simulink model "SMC_Boost4"  (R2016b)
settings: Solver=VariableStepAuto  StartTime=0.0  StopTime=0.1  RelTol=1e-3
libraries: powerlib x13
settings Model: Creator=mahdi  LastModifiedBy=mahdi

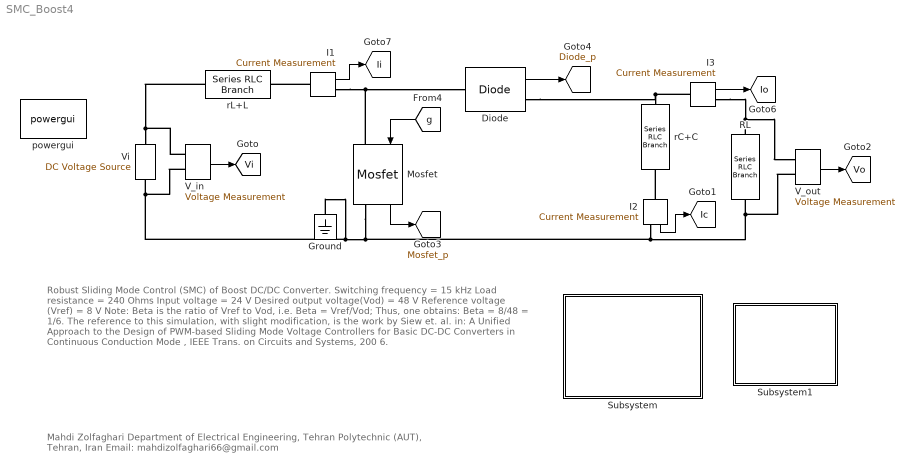
== system SMC_Boost4 ==
  note: Mahdi Zolfaghari
      | Department of Electrical Engineering, Tehran Polytechnic (AUT), Tehran, Iran
      | Email: mahdizolfaghari66@gmail.com
  note: Robust Sliding Mode Control (SMC) of Boost DC/DC Converter.
      | Switching frequency = 15 kHz
      | Load resistance = 240 Ohms
      | Input voltage = 24 V
      | Desired output voltage(Vod) = 48 V
      | Reference voltage (Vref) = 8 V
      | Note: Beta is the ratio of Vref to Vod, i.e. Beta = Vref/Vod; Thus, one obtains:
      | Beta = 8/48 = 1/6.
      | The reference to this simulation, with slight modification, is the work by Siew et. al. in:
      | A Unified Approach to the Design of PWM-based Sliding Mode Voltage Controllers
      | for Basic DC-DC Converters in Continuous Conduction Mode , IEEE Trans. on Circuits and Systems, 200 6.
  Diode : powerlib/Power Electronics/Diode  Ron=0.001  Lon=0  Vf=0.8  IC=0  UseSnubber=off  Rs=500  Cs=250e-9  Measurements=on
  Ground : powerlib/Elements/Ground  LConnTagsString=a
  I1 : powerlib/Measurements/Current Measurement  PhasorSimulation=off  OutputType=Complex  PSBequivalent=0
  I2 : powerlib/Measurements/Current Measurement  PhasorSimulation=off  OutputType=Complex  PSBequivalent=0
  I3 : powerlib/Measurements/Current Measurement  PhasorSimulation=off  OutputType=Complex  PSBequivalent=0
  Mosfet : powerlib/Power Electronics/Mosfet  Ron=0.1  Lon=0  Rd=0.01  Vfd=0  IC=0  Rs=1e5  Cs=inf  Measurements=on
  RL : powerlib/Elements/Series RLC Branch  LConnTagsString=__new0  RConnTagsString=__new0  BranchType=R  Resistance=240  Inductance=1e-3  SetiL0=off  InitialCurrent=0  Capacitance=0  Setx0=off  InitialVoltage=0  Measurements=None
  Subsystem : Subsystem
      mask Display: disp('Sliding Mode\nController')
  Subsystem1 : Subsystem
      mask Display: disp('Measurements')
  V_in : powerlib/Measurements/Voltage Measurement  PhasorSimulation=off  OutputType=Complex  PSBequivalent=0
  V_out : powerlib/Measurements/Voltage Measurement  PhasorSimulation=off  OutputType=Complex  PSBequivalent=0
  Vi : powerlib/Electrical Sources/DC Voltage Source  Amplitude=24  Measurements=None
  powergui : powerlib/powergui  Priority=1  SimulationMode=Discrete  SolverType=Tustin/Backward Euler (TBE)  SampleTime=50e-6  frequency=60  SPID=off  DisableSnubberDevices=off  DisableRonSwitches=off  DisableVfSwitches=off  SwTol=0  DisplayEquations=off  Interpol=off  ExternalGateDelay=off  methode=off  Ts=10  FunctionMessages=off  echomessages=off  HookPort=off  EnableUseOfTLC=off  x0status=blocks  frequencyindice=0  Pbase=100e6  ErrMax=1e-4  Iterations=50  UnitsV=kV  UnitsW=MW  buscounter=0  RestoreLinks=warning  ResistiveCurrentMeasurement=off  Frange=[0:2:500]  Ylog=off  Xlog=on  ShowGrid=off  save=off  variable=ZData  structure=0  ZoomFFT=off  StartTime=0.0  cycles=1  DisplayStyle=1  fundamental=60  FreqAxis=off  MaxFrequency=1000  frequencyindicesteady=1  RmsSteady=1  display=off
  rC+C : powerlib/Elements/Series RLC Branch  LConnTagsString=__new0  RConnTagsString=__new0  BranchType=RC  Resistance=69e-3  Inductance=1e-3  SetiL0=off  InitialCurrent=0  Capacitance=2300e-6  Setx0=off  InitialVoltage=0  Measurements=None
  rL+L : powerlib/Elements/Series RLC Branch  LConnTagsString=__new0  RConnTagsString=__new0  BranchType=RL  Resistance=0.14  Inductance=300e-6  SetiL0=off  InitialCurrent=0  Capacitance=0  Setx0=off  InitialVoltage=0  Measurements=None
  tag scope: Diode_p=global, Ic=global, Ii=global, Io=global, Mosfet_p=global, Vi=global, Vo=global
  wires:
  V_out/1 -> [Vo]
  I2/1 -> [Ic]
  V_in/1 -> [Vi]
  [g] -> Mosfet/1
  Mosfet/1 -> [Mosfet_p]
  Diode/1 -> [Diode_p]
  I3/1 -> [Io]
  I1/1 -> [Ii]
  connections:
  I2/LConn1 -- rC+C/RConn1
  RL/LConn1 -- I3/RConn1 -- V_out/LConn1
  rL+L/LConn1 -- V_in/LConn1 -- Vi/RConn1
  I2/RConn1 -- Ground/LConn1 -- V_in/LConn2 -- Vi/LConn1 -- Mosfet/RConn1 -- V_out/LConn2 -- RL/RConn1
  Diode/RConn1 -- rC+C/LConn1 -- I3/LConn1
  Mosfet/LConn1 -- I1/RConn1 -- Diode/LConn1
  I1/LConn1 -- rL+L/RConn1

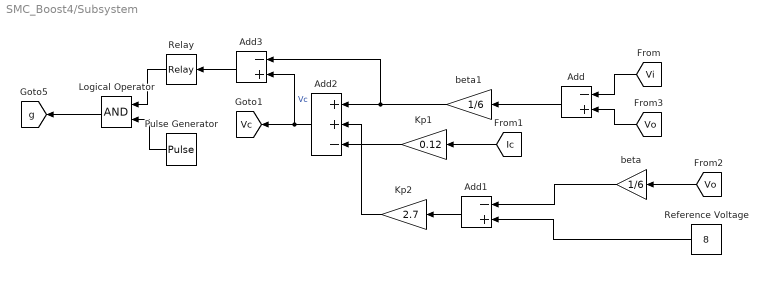
== system SMC_Boost4/Subsystem ==
  Add : Sum  Inputs=-+
  Add1 : Sum  Inputs=-+
  Add2 : Sum  Inputs=++-
  Add3 : Sum  Inputs=-+
  Kp1 : Gain  Gain=0.12
  Kp2 : Gain  Gain=2.7
  Logical Operator : Logic  AllPortsSameDT=off  OutDataTypeStr=boolean
  Pulse Generator : DiscretePulseGenerator  PulseType=Time based  Period=1/15e3  PulseWidth=50
  Reference Voltage : Constant  Value=8
  Relay : Relay  OnSwitchValue=3.75e-3  OffSwitchValue=3.5e-3
  beta : Gain  Gain=1/6
  beta1 : Gain  Gain=1/6
  tag scope: Vc=global, g=global
  wires:
  Add1/1 -> Kp2/1
  Add/1 -> beta1/1
  Relay/1 -> Logical Operator/1
  Pulse Generator/1 -> Logical Operator/2
  Logical Operator/1 -> [g]
  [Vi] -> Add/1
  Kp2/1 -> Add2/2
  Add3/1 -> Relay/1
  Add2/1 -> [Vc], Add3/2  "Vc"
  Reference Voltage/1 -> Add1/2
  beta/1 -> Add1/1
  Kp1/1 -> Add2/3
  [Vo] -> beta/1
  [Ic] -> Kp1/1
  beta1/1 -> Add3/1, Add2/1
  [Vo] -> Add/2

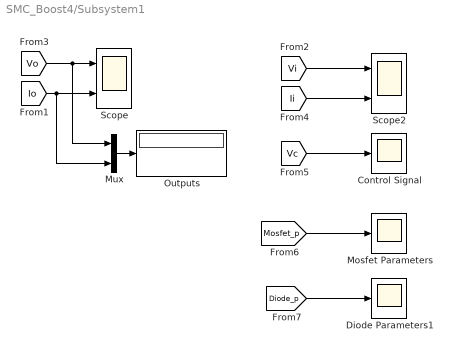
== system SMC_Boost4/Subsystem1 ==
  Control Signal : Scope
  Diode Parameters1 : Scope
  Mosfet Parameters : Scope
  Mux : Mux  Inputs=2
  Outputs : Display
  Scope : Scope  NumInputPorts=2
  Scope2 : Scope  NumInputPorts=2
  wires:
  Mux/1 -> Outputs/1
  [Vo] -> Mux/1, Scope/1
  [Io] -> Mux/2, Scope/2
  [Ii] -> Scope2/2
  [Vi] -> Scope2/1
  [Vc] -> Control Signal/1
  [Mosfet_p] -> Mosfet Parameters/1
  [Diode_p] -> Diode Parameters1/1
